simulink model "KanKimMiy91_r2018a"  (R2018a)
settings: Solver=ode45  StartTime=0.0  StopTime=4  RelTol=1e-5  EnableMultiTasking=on
undefined symbols (not defined in the file): KIm, Km, KPm, Pm
libraries: simulink x3
settings Model: Creator=dwbertol  LastModifiedBy=bruno
settings DataIOCC: LimitDataPoints=on  SaveFormat=Array  SignalLoggingSaveFormat=ModelDataLogs
settings OptimizationCC: ExpressionDepthLimit=2147483647  LifeSpan=inf
settings DebuggingCC: UnderspecifiedInitializationDetection=Classic  MergeDetectMultiDrivingBlocksExec=none  SolverPrmCheckMsg=warning  FcnCallInpInsideContextMsg=warning  StateNameClashWarn=warning  SFUnexpectedBacktrackingDiag=warning  SFNoUnconditionalDefaultTransitionDiag=warning  SFExecutionAtInitializationDiag=none
settings HardwareCC: ProdBitPerPointer=32  ProdBitPerSizeT=32  ProdBitPerPtrDiffT=32  ProdLargestAtomicFloat=None  ProdIntDivRoundTo=Undefined  ProdEndianess=Unspecified  ProdWordSize=32  ProdHWDeviceType=32-bit Generic
settings ModelReferenceCC: PropagateSignalLabelsOutOfModel=off
settings CodeAppCC: StateflowObjectComments=on
settings GRTTargetCC: TargetLangStandard=C89/C90 (ANSI)  GeneratePreprocessorConditionals=Disable all  CombineOutputUpdateFcns=off  GRTInterface=on
settings ConfigComp: CovMetricSettings=dw  CovHtmlReporting=on  CovSaveCumulativeToWorkspaceVar=on  CovSaveSingleToWorkspaceVar=on  CovExternalEMLEnable=off

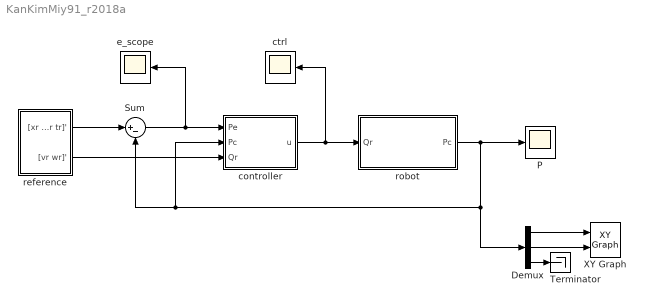
== system KanKimMiy91_r2018a ==
  Demux : Demux  Outputs=3
  P : Scope
  Sum : Sum  Inputs=|+-  AccumDataTypeStr=double
  Terminator : Terminator
  XY Graph : simulink/Sinks/XY Graph  xmin=-0.01  xmax=1  ymin=-0.01  ymax=0.1  st=-1
  controller : Subsystem  mask{kx=80, ky=2000, kt=160}
  ctrl : Scope
  e_scope : Scope
  reference : Subsystem  mask{vr=1, wr=0, ini=[0 0.02 0]}
  robot : Subsystem  mask{ini=[0 0 0]'}
  wires:
  controller/1(u) -> robot/1(Qr), ctrl/1
  Demux/3 -> Terminator/1
  Demux/2 -> XY Graph/2
  Demux/1 -> XY Graph/1
  reference/1("[xr yr tr]' ") -> Sum/1
  Sum/1 -> controller/1(Pe), e_scope/1
  reference/2("[vr wr]'") -> controller/3(Qr)
  robot/1(Pc) -> P/1, Demux/1, Sum/2, controller/2(Pc)

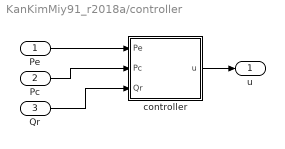
== system KanKimMiy91_r2018a/controller ==
  Pe : Inport
  Pc : Inport  Port=2
  Qr : Inport  Port=3
  controller : MATLAB Function  TreatAsAtomicUnit=on
  u : Outport
  wires:
  Qr/1 -> controller/3(Qr)
  Pc/1 -> controller/2(Pc)
  Pe/1 -> controller/1(Pe)
  controller/1(u) -> u/1

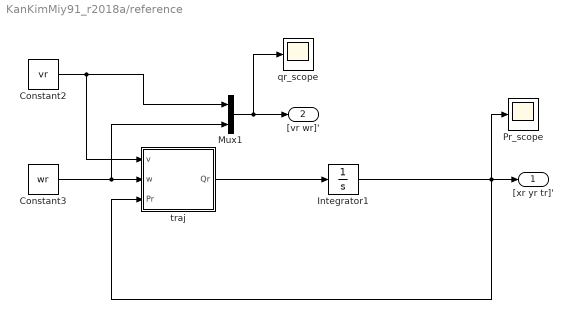
== system KanKimMiy91_r2018a/reference ==
  Constant2 : Constant  Value=vr  VectorParams1D=off
  Constant3 : Constant  Value=wr  VectorParams1D=off
  Integrator1 : Integrator  InitialCondition=ini
  Mux1 : Mux  Inputs=2
  Pr_scope : Scope
  qr_scope : Scope
  traj : MATLAB Function  TreatAsAtomicUnit=on
  "[xr yr tr]' " : Outport
  "[vr wr]'" : Outport  Port=2
  wires:
  Constant2/1 -> traj/1(v), Mux1/1
  Mux1/1 -> "[vr wr]'"/1, qr_scope/1
  traj/1(Qr) -> Integrator1/1
  Constant3/1 -> Mux1/2, traj/2(w)
  Integrator1/1 -> Pr_scope/1, traj/3(Pr), "[xr yr tr]' "/1

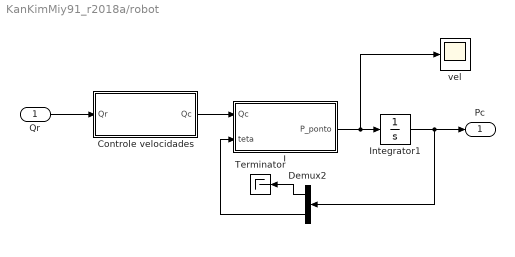
== system KanKimMiy91_r2018a/robot ==
  Qr : Inport
  Controle velocidades : Subsystem
  Demux2 : Demux  Outputs=[2 1]
  Integrator1 : Integrator  InitialCondition=ini
  J : MATLAB Function  TreatAsAtomicUnit=on
  Terminator : Terminator
  vel : Scope
  Pc : Outport
  wires:
  J/1(P_ponto) -> vel/1, Integrator1/1
  Integrator1/1 -> Demux2/1, Pc/1
  Demux2/1 -> Terminator/1
  Qr/1 -> Controle velocidades/1(Qr)
  Controle velocidades/1(Qc) -> J/1(Qc)
  Demux2/2 -> J/2(teta)

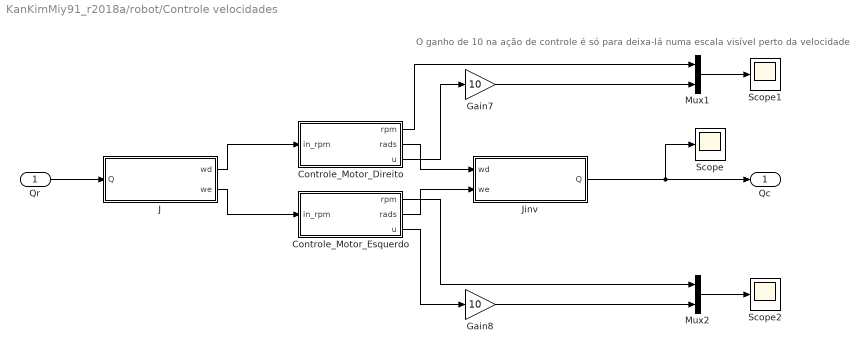
== system KanKimMiy91_r2018a/robot/Controle velocidades ==
  note: O ganho de 10 na ação de controle é só para deixa-lá numa escala visível perto da velocidade
  Qr : Inport
  Controle_Motor_Direito : Subsystem
  Controle_Motor_Esquerdo : Subsystem
  Gain7 : Gain  Gain=10
  Gain8 : Gain  Gain=10
  J : MATLAB Function  TreatAsAtomicUnit=on
  Jinv : MATLAB Function  TreatAsAtomicUnit=on
  Mux1 : Mux  Inputs=2
  Mux2 : Mux  Inputs=2
  Scope : Scope
  Scope1 : Scope
  Scope2 : Scope
  Qc : Outport
  wires:
  Gain7/1 -> Mux1/2
  Mux2/1 -> Scope2/1
  Mux1/1 -> Scope1/1
  Gain8/1 -> Mux2/2
  Controle_Motor_Direito/3(u) -> Gain7/1
  Controle_Motor_Direito/1(rpm) -> Mux1/1
  Controle_Motor_Esquerdo/3(u) -> Gain8/1
  Controle_Motor_Esquerdo/1(rpm) -> Mux2/1
  Qr/1 -> J/1(Q)
  J/1(wd) -> Controle_Motor_Direito/1(in_rpm)
  J/2(we) -> Controle_Motor_Esquerdo/1(in_rpm)
  Controle_Motor_Direito/2(rads) -> Jinv/1(wd)
  Controle_Motor_Esquerdo/2(rads) -> Jinv/2(we)
  Jinv/1(Q) -> Scope/1, Qc/1

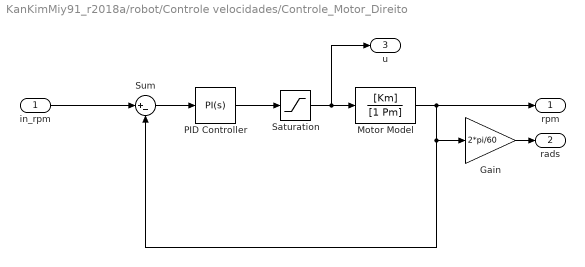
== system KanKimMiy91_r2018a/robot/Controle velocidades/Controle_Motor_Direito ==
  in_rpm : Inport
  Gain : Gain  Gain=2*pi/60
  Motor Model : TransferFcn  Numerator=[Km]  Denominator=[1 Pm]
  PID Controller : simulink/Continuous/PID Controller  Controller=PI  TimeDomain=Continuous-time  SampleTime=-1  IntegratorMethod=Forward Euler  FilterMethod=Forward Euler  Form=Parallel  UseFilter=on  ControllerParametersSource=internal  P=KPm  I=KIm  D=0  N=0  InitialConditionSource=internal  InitialConditionForIntegrator=0  InitialConditionForFilter=0  ExternalReset=none  LimitOutput=off  UpperSaturationLimit=inf  LowerSaturationLimit=-inf  LinearizeAsGain=on  AntiWindupMode=none  Kb=1  TrackingMode=off  Kt=1  PParamMin=[]  PParamMax=[]  IParamMin=[]  IParamMax=[]  DParamMin=[]  DParamMax=[]  NParamMin=[]  NParamMax=[]  KbParamMin=[]  KbParamMax=[]  KtParamMin=[]  KtParamMax=[]  POutMin=[]  POutMax=[]  IOutMin=[]  IOutMax=[]  DOutMin=[]  DOutMax=[]  NOutMin=[]  NOutMax=[]  KbOutMin=[]  KbOutMax=[]  KtOutMin=[]  KtOutMax=[]  IntegratorOutMin=[]  IntegratorOutMax=[]  FilterOutMin=[]  FilterOutMax=[]  SumOutMin=[]  SumOutMax=[]  SumI1OutMin=[]  SumI1OutMax=[]  SumI2OutMin=[]  SumI2OutMax=[]  SumI3OutMin=[]  SumI3OutMax=[]  SumDOutMin=[]  SumDOutMax=[]  SaturationOutMin=[]  SaturationOutMax=[]  IntegratorContinuousStateAttributes=''  IntegratorStateMustResolveToSignalObject=off  IntegratorRTWStateStorageClass=Auto  FilterContinuousStateAttributes=''  FilterStateMustResolveToSignalObject=off  FilterRTWStateStorageClass=Auto  DifferentiatorICPrevScaledInput=0  DifferentiatorOutMin=[]  DifferentiatorOutMax=[]  FilterDiffOutCoefMin=[]  FilterDiffOutCoefMax=[]  SumDenOutMin=[]  SumDenOutMax=[]  SumNumOutMin=[]  SumNumOutMax=[]  ReciprocalOutMin=[]  ReciprocalOutMax=[]  DivideOutMin=[]  DivideOutMax=[]  TunerSelectOption=Transfer Function Based (PID Tuner App)
  Saturation : Saturate  UpperLimit=100  LowerLimit=-100
  Sum : Sum  Inputs=|+-
  rpm : Outport
  rads : Outport  Port=2
  u : Outport  Port=3
  wires:
  PID Controller/1 -> Saturation/1
  Motor Model/1 -> rpm/1, Gain/1, Sum/2
  Saturation/1 -> u/1, Motor Model/1
  Sum/1 -> PID Controller/1
  in_rpm/1 -> Sum/1
  Gain/1 -> rads/1

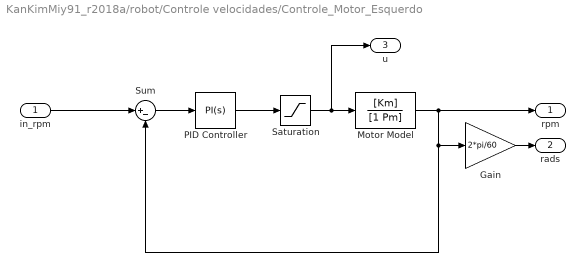
== system KanKimMiy91_r2018a/robot/Controle velocidades/Controle_Motor_Esquerdo ==
  in_rpm : Inport
  Gain : Gain  Gain=2*pi/60
  Motor Model : TransferFcn  Numerator=[Km]  Denominator=[1 Pm]
  PID Controller : simulink/Continuous/PID Controller  Controller=PI  TimeDomain=Continuous-time  SampleTime=-1  IntegratorMethod=Forward Euler  FilterMethod=Forward Euler  Form=Parallel  UseFilter=on  ControllerParametersSource=internal  P=KPm  I=KIm  D=0  N=0  InitialConditionSource=internal  InitialConditionForIntegrator=0  InitialConditionForFilter=0  ExternalReset=none  LimitOutput=off  UpperSaturationLimit=inf  LowerSaturationLimit=-inf  LinearizeAsGain=on  AntiWindupMode=none  Kb=1  TrackingMode=off  Kt=1  PParamMin=[]  PParamMax=[]  IParamMin=[]  IParamMax=[]  DParamMin=[]  DParamMax=[]  NParamMin=[]  NParamMax=[]  KbParamMin=[]  KbParamMax=[]  KtParamMin=[]  KtParamMax=[]  POutMin=[]  POutMax=[]  IOutMin=[]  IOutMax=[]  DOutMin=[]  DOutMax=[]  NOutMin=[]  NOutMax=[]  KbOutMin=[]  KbOutMax=[]  KtOutMin=[]  KtOutMax=[]  IntegratorOutMin=[]  IntegratorOutMax=[]  FilterOutMin=[]  FilterOutMax=[]  SumOutMin=[]  SumOutMax=[]  SumI1OutMin=[]  SumI1OutMax=[]  SumI2OutMin=[]  SumI2OutMax=[]  SumI3OutMin=[]  SumI3OutMax=[]  SumDOutMin=[]  SumDOutMax=[]  SaturationOutMin=[]  SaturationOutMax=[]  IntegratorContinuousStateAttributes=''  IntegratorStateMustResolveToSignalObject=off  IntegratorRTWStateStorageClass=Auto  FilterContinuousStateAttributes=''  FilterStateMustResolveToSignalObject=off  FilterRTWStateStorageClass=Auto  DifferentiatorICPrevScaledInput=0  DifferentiatorOutMin=[]  DifferentiatorOutMax=[]  FilterDiffOutCoefMin=[]  FilterDiffOutCoefMax=[]  SumDenOutMin=[]  SumDenOutMax=[]  SumNumOutMin=[]  SumNumOutMax=[]  ReciprocalOutMin=[]  ReciprocalOutMax=[]  DivideOutMin=[]  DivideOutMax=[]  TunerSelectOption=Transfer Function Based (PID Tuner App)
  Saturation : Saturate  UpperLimit=100  LowerLimit=-100
  Sum : Sum  Inputs=|+-
  rpm : Outport
  rads : Outport  Port=2
  u : Outport  Port=3
  wires:
  PID Controller/1 -> Saturation/1
  Saturation/1 -> u/1, Motor Model/1
  Sum/1 -> PID Controller/1
  in_rpm/1 -> Sum/1
  Motor Model/1 -> rpm/1, Gain/1, Sum/2
  Gain/1 -> rads/1

== matlab function KanKimMiy91_r2018a/reference/traj ==
  data: v input; w input; Pr input; Qr output
function Qr = fcn(v, w, Pr)

 Qr = [cos(Pr(3)) 0; sin(Pr(3)) 0; 0 1]*[v; w];
 
end

== matlab function KanKimMiy91_r2018a/robot/Controle velocidades/J ==
  data: Q input; wd output; we output
function [wd, we] = fcn(Q)
% Dados do robô
r = 16e-3;      % Raio da roda
a = 69e-3;      % Distância do centro do robô até o centro das rodas

w_mot_rpm = (60/(2*pi))*[1/r a/r; 1/r -a/r]*Q;   % o 60/(2pi) é pra converter p/ rpm
wd = w_mot_rpm(1);
we = w_mot_rpm(2);

== matlab function KanKimMiy91_r2018a/robot/Controle velocidades/Jinv ==
  data: wd input; Q output; we input
function Q = fcn(wd, we)
% Dados do robô
r = 16e-3;      % Raio da roda
a = 69e-3;      % Distância do centro do robô até o centro das rodas

Q = (r/2)*[1 1; 1/a -1/a]*[wd; we];

== matlab function KanKimMiy91_r2018a/controller/controller ==
  data: Pe input; Pc input; Qr input; u output; kx parameter; ky parameter; kt parameter
function u = fcn(Pe,Pc,Qr,kx,ky,kt)

 Pe = [cos(Pc(3)) sin(Pc(3)) 0; -sin(Pc(3)) cos(Pc(3)) 0; 0 0 1]*Pe;
%  Pe(1) = 0;  %essa linha é um caso a parte (para o seguidor de linha)
 u = [Qr(1)*cos(Pe(3))+kx*Pe(1) Qr(2)+Qr(1)*(ky*Pe(2)+kt*sin(Pe(3)))]';
 
end

== matlab function KanKimMiy91_r2018a/robot/J ==
  data: Qc input; P_ponto output; teta input
function P_ponto = fcn(Qc, teta)

P_ponto = [Qc(1)*cos(teta); Qc(1)*sin(teta); Qc(2)]; %[Vx, Vy, Vteta];
